simulink model "jamesWebb"  (R2024a)
settings: Solver=FixedStepAuto  StartTime=0.0  StopTime=63072000  FixedStep=100  RelTol=1e-3
values from neighbouring files (symbols this model uses):
  G = 6.674e-11    [JamesWebbSim.m]
  mE = 5.97219e24    (= 5.97219e+24)    [JamesWebbSim.m]
  mS = 1988410e24    (= 1.98841e+30)    [JamesWebbSim.m]
  posE = [-5.270751030639560E+07 -1.424211399657750E+08 3.602153098984063E+04]*1000    [JamesWebbSim.m]
  posJ = [-5.256168304341657E+07 -1.440483280181565E+08 -1.734837072574794E+05]*1000    [JamesWebbSim.m]
  velE = [2.755293933513340E+01 -1.021705234088606E+01 -3.346080722117506E-04]*1000    [JamesWebbSim.m]
  velJ = [2.771985965841215E+01 -1.024983981129689E+01 -1.464231284627822E-01]*1000    [JamesWebbSim.m]
settings Model: Creator=User  LastModifiedBy=User

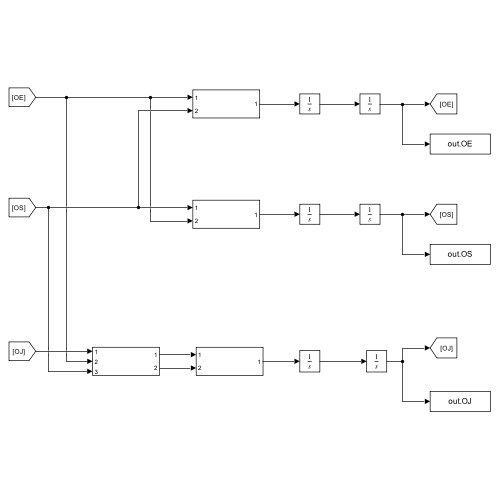
[thumbnail: Simulink's stored preview of the top-level diagram]
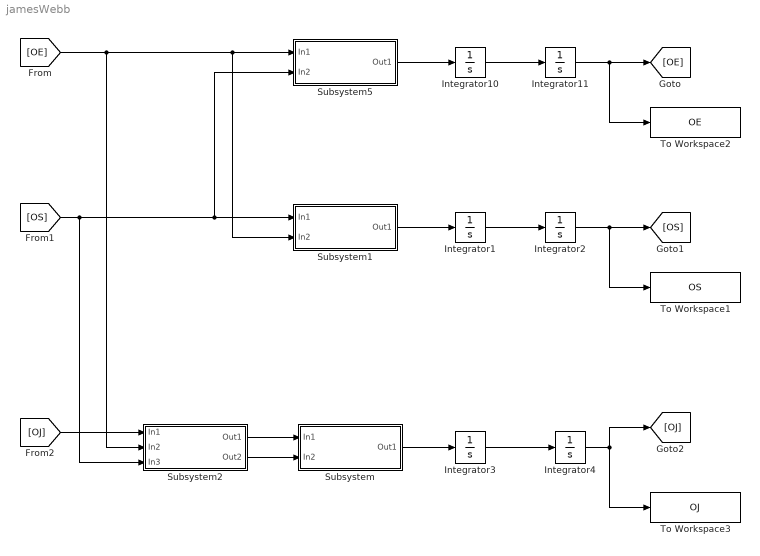
== system jamesWebb ==
  Integrator1 : Integrator
  Integrator10 : Integrator  InitialCondition=velE
  Integrator11 : Integrator  InitialCondition=posE
  Integrator2 : Integrator
  Integrator3 : Integrator  InitialCondition=velJ
  Integrator4 : Integrator  InitialCondition=posJ
  Subsystem : Subsystem
  Subsystem1 : Subsystem
  Subsystem2 : Subsystem
  Subsystem5 : Subsystem
  To Workspace1 : ToWorkspace  VariableName=OS  SaveFormat=Timeseries  SampleTime=-1
  To Workspace2 : ToWorkspace  VariableName=OE  SaveFormat=Timeseries  SampleTime=-1
  To Workspace3 : ToWorkspace  VariableName=OJ  SaveFormat=Timeseries  SampleTime=-1
  wires:
  Integrator10/1 -> Integrator11/1
  [OS] -> Subsystem2/3(In3), Subsystem1/1(In1), Subsystem5/2(In2)
  Integrator11/1 -> To Workspace2/1, [OE]
  Subsystem2/2(Out2) -> Subsystem/2(In2)
  Integrator2/1 -> To Workspace1/1, [OS]
  [OE] -> Subsystem2/2(In2), Subsystem1/2(In2), Subsystem5/1(In1)
  Subsystem5/1(Out1) -> Integrator10/1
  Integrator4/1 -> To Workspace3/1, [OJ]
  Subsystem2/1(Out1) -> Subsystem/1(In1)
  Integrator1/1 -> Integrator2/1
  Integrator3/1 -> Integrator4/1
  [OJ] -> Subsystem2/1(In1)
  Subsystem1/1(Out1) -> Integrator1/1
  Subsystem/1(Out1) -> Integrator3/1

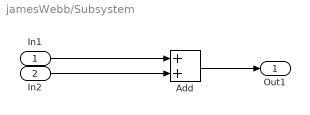
== system jamesWebb/Subsystem ==
  In1 : Inport
  In2 : Inport  Port=2
  Add : Sum
  Out1 : Outport
  wires:
  Add/1 -> Out1/1
  In1/1 -> Add/1
  In2/1 -> Add/2

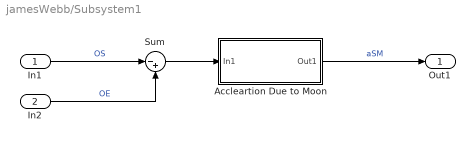
== system jamesWebb/Subsystem1 ==
  In1 : Inport
  In2 : Inport  Port=2
  Accleartion Due to Moon : Subsystem
  Sum : Sum  Inputs=|-+
  Out1 : Outport
  wires:
  Accleartion Due to Moon/1(Out1) -> Out1/1  "aSM"
  Sum/1 -> Accleartion Due to Moon/1(In1)
  In1/1 -> Sum/1  "OS"
  In2/1 -> Sum/2  "OE"

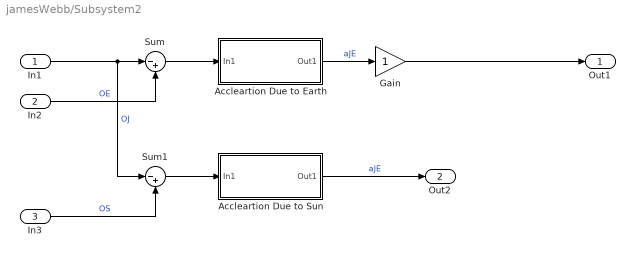
== system jamesWebb/Subsystem2 ==
  In1 : Inport
  In2 : Inport  Port=2
  In3 : Inport  Port=3
  Accleartion Due to Earth : Subsystem
  Accleartion Due to Sun : Subsystem
  Gain : Gain
  Sum : Sum  Inputs=|-+
  Sum1 : Sum  Inputs=|-+
  Out1 : Outport
  Out2 : Outport  Port=2
  wires:
  Accleartion Due to Earth/1(Out1) -> Gain/1  "aJE"
  Sum/1 -> Accleartion Due to Earth/1(In1)
  In1/1 -> Sum1/1, Sum/1  "OJ"
  In2/1 -> Sum/2  "OE"
  Sum1/1 -> Accleartion Due to Sun/1(In1)
  Accleartion Due to Sun/1(Out1) -> Out2/1  "aJE"
  In3/1 -> Sum1/2  "OS"
  Gain/1 -> Out1/1

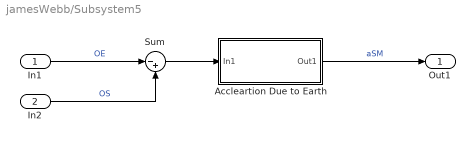
== system jamesWebb/Subsystem5 ==
  In1 : Inport
  In2 : Inport  Port=2
  Accleartion Due to Earth : Subsystem
  Sum : Sum  Inputs=|-+
  Out1 : Outport
  wires:
  Accleartion Due to Earth/1(Out1) -> Out1/1  "aSM"
  Sum/1 -> Accleartion Due to Earth/1(In1)
  In1/1 -> Sum/1  "OE"
  In2/1 -> Sum/2  "OS"

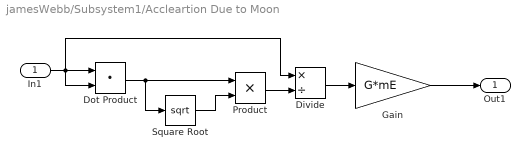
== system jamesWebb/Subsystem1/Accleartion Due to Moon ==
  In1 : Inport
  Divide : Product  Inputs=*/
  Dot Product : DotProduct  OutDataTypeStr=Inherit: Inherit via internal rule
  Gain : Gain  Gain=G*mE
  Product : Product
  Square Root : Sqrt
  Out1 : Outport
  wires:
  In1/1 -> Divide/1, Dot Product/2, Dot Product/1
  Dot Product/1 -> Square Root/1, Product/1
  Square Root/1 -> Product/2
  Product/1 -> Divide/2
  Gain/1 -> Out1/1
  Divide/1 -> Gain/1

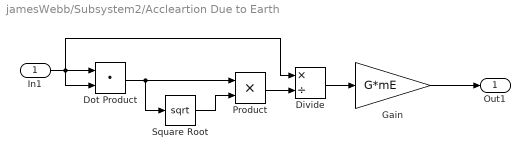
== system jamesWebb/Subsystem2/Accleartion Due to Earth ==
  In1 : Inport
  Divide : Product  Inputs=*/
  Dot Product : DotProduct  OutDataTypeStr=Inherit: Inherit via internal rule
  Gain : Gain  Gain=G*mE
  Product : Product
  Square Root : Sqrt
  Out1 : Outport
  wires:
  In1/1 -> Divide/1, Dot Product/2, Dot Product/1
  Dot Product/1 -> Square Root/1, Product/1
  Square Root/1 -> Product/2
  Product/1 -> Divide/2
  Gain/1 -> Out1/1
  Divide/1 -> Gain/1

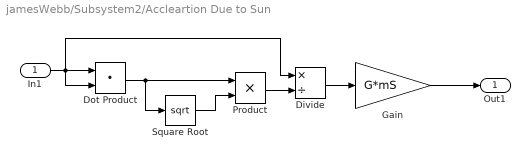
== system jamesWebb/Subsystem2/Accleartion Due to Sun ==
  In1 : Inport
  Divide : Product  Inputs=*/
  Dot Product : DotProduct  OutDataTypeStr=Inherit: Inherit via internal rule
  Gain : Gain  Gain=G*mS
  Product : Product
  Square Root : Sqrt
  Out1 : Outport
  wires:
  In1/1 -> Divide/1, Dot Product/2, Dot Product/1
  Dot Product/1 -> Square Root/1, Product/1
  Square Root/1 -> Product/2
  Product/1 -> Divide/2
  Gain/1 -> Out1/1
  Divide/1 -> Gain/1

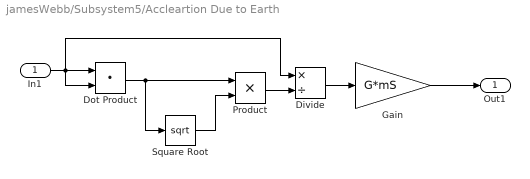
== system jamesWebb/Subsystem5/Accleartion Due to Earth ==
  In1 : Inport
  Divide : Product  Inputs=*/
  Dot Product : DotProduct  OutDataTypeStr=Inherit: Inherit via internal rule
  Gain : Gain  Gain=G*mS
  Product : Product
  Square Root : Sqrt
  Out1 : Outport
  wires:
  In1/1 -> Divide/1, Dot Product/2, Dot Product/1
  Dot Product/1 -> Square Root/1, Product/1
  Square Root/1 -> Product/2
  Product/1 -> Divide/2
  Gain/1 -> Out1/1
  Divide/1 -> Gain/1
